simulink model "sim3"  (R2023b)
settings: Solver=ode45  StartTime=0.0  StopTime=10.0  RelTol=1e-3
undefined symbols (not defined in the file): Beq, Bp, Fc, g, Ip, Lp, Mc, Mp
settings Model: Creator=dayan  LastModifiedBy=dayan

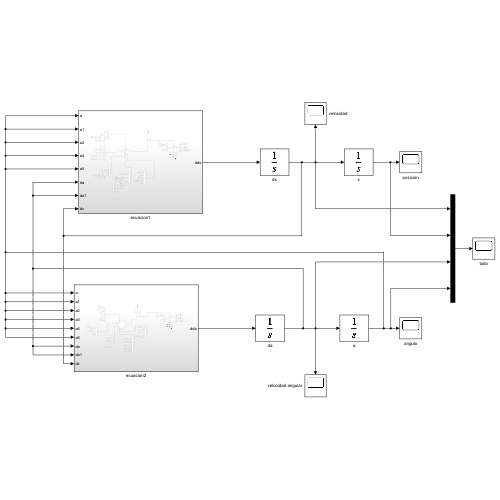
[thumbnail: Simulink's stored preview of the top-level diagram]
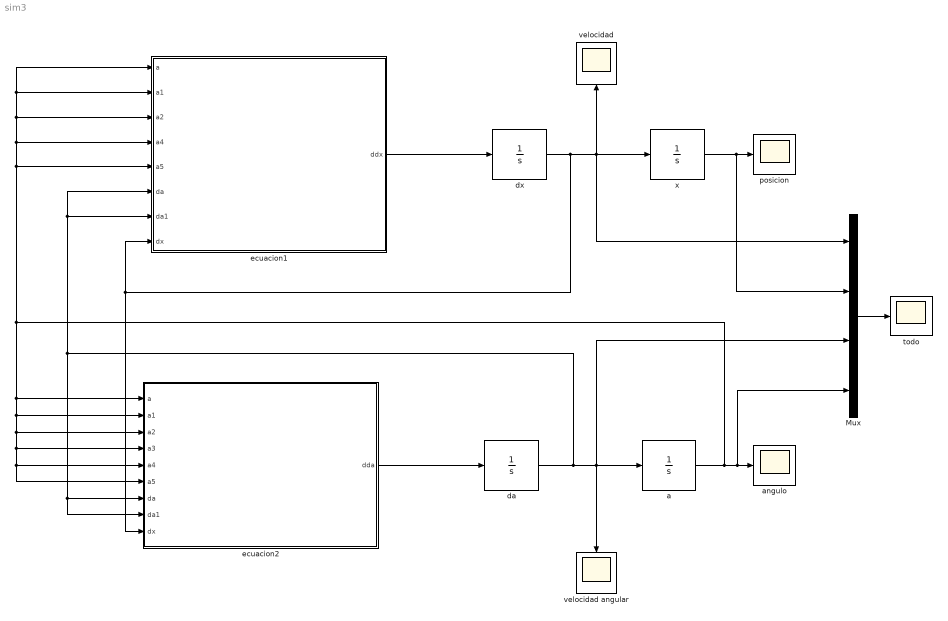
== system sim3 ==
  Mux : Mux
  a : Integrator  InitialCondition=0.017
  angulo : Scope
  da : Integrator
  dx : Integrator
  ecuacion1 : Subsystem
  ecuacion2 : Subsystem
  posicion : Scope
  todo : Scope
  velocidad : Scope
  velocidad angular : Scope
  x : Integrator
  wires:
  dx/1 -> ecuacion2/9(dx), ecuacion1/8(dx), velocidad/1, Mux/1, x/1
  ecuacion1/1(ddx) -> dx/1
  ecuacion2/1(dda) -> da/1
  da/1 -> ecuacion2/7(da), ecuacion2/8(da1), ecuacion1/7(da1), ecuacion1/6(da), velocidad angular/1, Mux/3, a/1
  a/1 -> ecuacion2/1(a), ecuacion2/2(a1), ecuacion2/3(a2), ecuacion2/4(a3), ecuacion2/5(a4), ecuacion2/6(a5), ecuacion1/5(a5), ecuacion1/4(a4), ecuacion1/3(a2), ecuacion1/2(a1), ecuacion1/1(a), Mux/4, angulo/1
  x/1 -> Mux/2, posicion/1
  Mux/1 -> todo/1

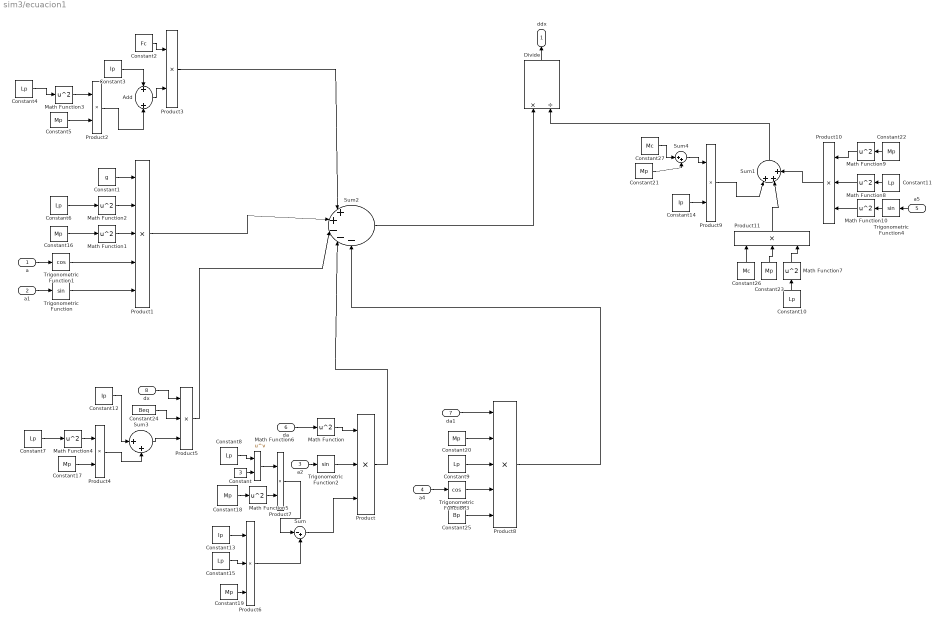
== system sim3/ecuacion1 ==
  a : Inport
  a1 : Inport  Port=2
  a2 : Inport  Port=3
  a4 : Inport  Port=4
  a5 : Inport  Port=5
  da : Inport  Port=6
  da1 : Inport  Port=7
  dx : Inport  Port=8
  Add : Sum
  Constant : Constant  Value=3
  Constant1 : Constant  Value=g
  Constant{4,6..11,15} (8 alike) : Constant  Value=Lp
  Constant{3,12..14} (4 alike) : Constant  Value=Ip
  Constant{5,16..23} (9 alike) : Constant  Value=Mp  VectorParams1D=off  SampleTime=-1
  Constant2 : Constant  Value=Fc
  Constant24 : Constant  Value=Beq
  Constant25 : Constant  Value=Bp
  Constant26 : Constant  Value=Mc
  Constant27 : Constant  Value=Mc
  Divide : Product  Inputs=*/
  Math Function{,1..5,7..10} (10 alike) : Math  Operator=square
  Math Function6 : Math  Operator=pow
  Product{,5..6,10..11} (5 alike) : Product  Inputs=3
  Product1 : Product  Inputs=5
  Product{2..4,7,9} (5 alike) : Product
  Product8 : Product  Inputs=5
  Sum : Sum  Inputs=|-+
  Sum1 : Sum  Inputs=|+++
  Sum2 : Sum  Inputs=|++---
  Sum3 : Sum  Inputs=|++
  Sum4 : Sum  Inputs=|++
  Trigonometric Function : Trigonometry
  Trigonometric Function1 : Trigonometry  Operator=cos
  Trigonometric Function2 : Trigonometry
  Trigonometric Function3 : Trigonometry  Operator=cos
  Trigonometric Function4 : Trigonometry
  ddx : Outport
  wires:
  Constant2/1 -> Product3/1
  Constant5/1 -> Product2/2
  Product2/1 -> Add/2
  Product3/1 -> Sum2/1
  Constant3/1 -> Add/1
  Math Function3/1 -> Product2/1
  Constant4/1 -> Math Function3/1
  Add/1 -> Product3/2
  Math Function2/1 -> Product1/2
  Constant6/1 -> Math Function2/1
  Product1/1 -> Sum2/2
  Trigonometric Function/1 -> Product1/5
  Constant1/1 -> Product1/1
  Trigonometric Function1/1 -> Product1/4
  Constant16/1 -> Math Function1/1
  Math Function1/1 -> Product1/3
  Sum3/1 -> Product5/3
  Product5/1 -> Sum2/3
  Math Function4/1 -> Product4/1
  Constant17/1 -> Product4/2
  Product4/1 -> Sum3/2
  Constant12/1 -> Sum3/1
  Constant7/1 -> Math Function4/1
  Trigonometric Function2/1 -> Product/2
  Constant18/1 -> Math Function5/1
  Math Function6/1 -> Product7/1
  Sum/1 -> Product/3
  a2/1 -> Trigonometric Function2/1
  Math Function5/1 -> Product7/2
  Math Function/1 -> Product/1
  Constant/1 -> Math Function6/2
  Constant13/1 -> Product6/1
  Product7/1 -> Sum/1
  Constant8/1 -> Math Function6/1
  Constant19/1 -> Product6/3
  Product6/1 -> Sum/2
  Constant25/1 -> Product8/5
  Trigonometric Function3/1 -> Product8/4
  Constant9/1 -> Product8/3
  Constant20/1 -> Product8/2
  a5/1 -> Trigonometric Function4/1
  Math Function7/1 -> Product11/3
  Product9/1 -> Sum1/1
  Product10/1 -> Sum1/3
  Math Function8/1 -> Product10/2
  Constant11/1 -> Math Function8/1
  Sum4/1 -> Product9/1
  Constant26/1 -> Product11/1
  Constant23/1 -> Product11/2
  Product11/1 -> Sum1/2
  Constant22/1 -> Math Function9/1
  Constant10/1 -> Math Function7/1
  Constant27/1 -> Sum4/1
  Math Function9/1 -> Product10/1
  Product/1 -> Sum2/4
  Product8/1 -> Sum2/5
  Sum2/1 -> Divide/1
  Sum1/1 -> Divide/2
  a/1 -> Trigonometric Function1/1
  a1/1 -> Trigonometric Function/1
  dx/1 -> Product5/1
  da/1 -> Math Function/1
  a4/1 -> Trigonometric Function3/1
  da1/1 -> Product8/1
  Divide/1 -> ddx/1
  Constant14/1 -> Product9/2
  Constant15/1 -> Product6/2
  Constant21/1 -> Sum4/2
  Constant24/1 -> Product5/2
  Math Function10/1 -> Product10/3
  Trigonometric Function4/1 -> Math Function10/1

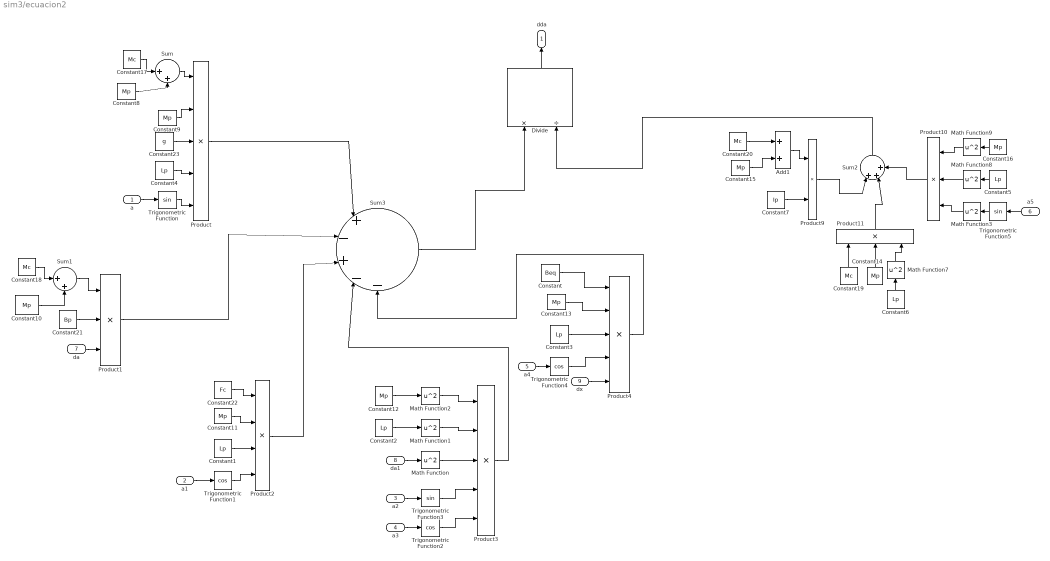
== system sim3/ecuacion2 ==
  a : Inport
  a1 : Inport  Port=2
  a2 : Inport  Port=3
  a3 : Inport  Port=4
  a4 : Inport  Port=5
  a5 : Inport  Port=6
  da : Inport  Port=7
  da1 : Inport  Port=8
  dx : Inport  Port=9
  Add1 : Sum
  Constant : Constant  Value=Beq
  Constant{1..6} (6 alike) : Constant  Value=Lp
  Constant{8..16} (9 alike) : Constant  Value=Mp  VectorParams1D=off  SampleTime=-1
  Constant{17..20} (4 alike) : Constant  Value=Mc
  Constant21 : Constant  Value=Bp
  Constant22 : Constant  Value=Fc
  Constant23 : Constant  Value=g
  Constant7 : Constant  Value=Ip
  Divide : Product  Inputs=*/
  Math Function{,1..3,7..9} (7 alike) : Math  Operator=square
  Product : Product  Inputs=5
  Product1 : Product  Inputs=3
  Product10 : Product  Inputs=3
  Product11 : Product  Inputs=3
  Product2 : Product  Inputs=4
  Product3 : Product  Inputs=5
  Product4 : Product  Inputs=5
  Product9 : Product
  Sum : Sum  Inputs=|++
  Sum1 : Sum  Inputs=|++
  Sum2 : Sum  Inputs=|+++
  Sum3 : Sum  Inputs=|+-+--
  Trigonometric Function : Trigonometry
  Trigonometric Function1 : Trigonometry  Operator=cos
  Trigonometric Function2 : Trigonometry  Operator=cos
  Trigonometric Function3 : Trigonometry
  Trigonometric Function4 : Trigonometry  Operator=cos
  Trigonometric Function5 : Trigonometry
  dda : Outport
  wires:
  Constant17/1 -> Sum/1
  Constant4/1 -> Product/4
  Sum/1 -> Product/1
  Constant23/1 -> Product/3
  Trigonometric Function/1 -> Product/5
  Constant9/1 -> Product/2
  Constant10/1 -> Sum1/2
  Sum1/1 -> Product1/1
  Constant21/1 -> Product1/2
  Product1/1 -> Sum3/2
  Constant18/1 -> Sum1/1
  Trigonometric Function1/1 -> Product2/4
  Constant1/1 -> Product2/3
  Constant11/1 -> Product2/2
  Product2/1 -> Sum3/3
  Product3/1 -> Sum3/4
  Math Function1/1 -> Product3/2
  Math Function2/1 -> Product3/1
  Trigonometric Function3/1 -> Product3/4
  Constant2/1 -> Math Function1/1
  Trigonometric Function2/1 -> Product3/5
  Constant12/1 -> Math Function2/1
  Math Function/1 -> Product3/3
  Product4/1 -> Sum3/5
  Constant13/1 -> Product4/2
  Constant3/1 -> Product4/3
  Trigonometric Function4/1 -> Product4/4
  Sum2/1 -> Divide/2
  Constant6/1 -> Math Function7/1
  Product11/1 -> Sum2/2
  Math Function8/1 -> Product10/2
  Product9/1 -> Sum2/1
  Constant14/1 -> Product11/2
  Add1/1 -> Product9/1
  Product10/1 -> Sum2/3
  Math Function7/1 -> Product11/3
  Constant5/1 -> Math Function8/1
  Math Function9/1 -> Product10/1
  Product/1 -> Sum3/1
  Sum3/1 -> Divide/1
  a/1 -> Trigonometric Function/1
  da/1 -> Product1/3
  a1/1 -> Trigonometric Function1/1
  a2/1 -> Trigonometric Function3/1
  da1/1 -> Math Function/1
  a3/1 -> Trigonometric Function2/1
  a4/1 -> Trigonometric Function4/1
  dx/1 -> Product4/5
  a5/1 -> Trigonometric Function5/1
  Divide/1 -> dda/1
  Constant7/1 -> Product9/2
  Constant8/1 -> Sum/2
  Constant15/1 -> Add1/2
  Constant16/1 -> Math Function9/1
  Constant/1 -> Product4/1
  Constant19/1 -> Product11/1
  Constant20/1 -> Add1/1
  Constant22/1 -> Product2/1
  Math Function3/1 -> Product10/3
  Trigonometric Function5/1 -> Math Function3/1
